simulink subsystem "State_Machine_S1"  (R2023b)
settings: Solver=VariableStepAuto  StartTime=0.0  StopTime=10.0  RelTol=1e-3
undefined symbols (not defined in the file): lb, nF, ub
libraries: dspstat3 x1
settings Model: Creator=Inver  LastModifiedBy=Inver

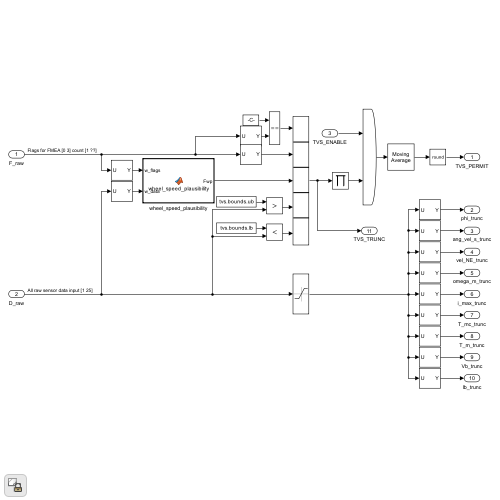
[thumbnail: Simulink's stored preview of the top-level diagram]
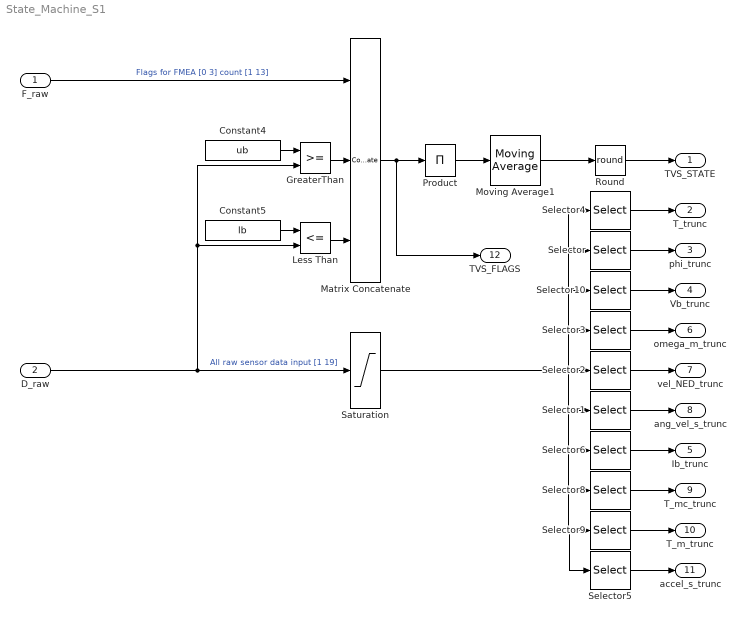
== system State_Machine_S1 ==
  F_raw : Inport
  D_raw : Inport  Port=2
  Constant4 : Constant  Value=ub
  Constant5 : Constant  Value=lb
  GreaterThan : RelationalOperator  OutDataTypeStr=boolean  RndMeth=Simplest  InputSameDT=off
  Less Than : RelationalOperator  Operator=<=  OutDataTypeStr=boolean  RndMeth=Simplest  InputSameDT=off
  Matrix Concatenate : Concatenate  NumInputs=3  ConcatenateDimension=2
  Moving Average1 : dspstat3/Moving Average  Method=Sliding window  ForgettingFactorPort=off  SpecifyWindowLength=on  WindowLength=nF  OverlapLength=nF-1  AllowArbitraryInputLength=off  ForgettingFactor=0.9  SimulateUsing=Code generation
  Product : Product  Inputs=1  OutDataTypeStr=double  SaturateOnIntegerOverflow=on
  Round : Rounding  Operator=round
  Saturation : Saturate  UpperLimit=ub  LowerLimit=lb
  Selector : Selector  IndexMode=Zero-based  InputPortWidth=19  IndexOptions=Index vector (dialog)  Indices=1  OutputSizes=1
  Selector1 : Selector  IndexMode=Zero-based  InputPortWidth=19  IndexOptions=Index vector (dialog)  Indices=[8 9 10]  OutputSizes=1
  Selector10 : Selector  IndexMode=Zero-based  InputPortWidth=19  IndexOptions=Index vector (dialog)  Indices=2  OutputSizes=1
  Selector2 : Selector  IndexMode=Zero-based  InputPortWidth=19  IndexOptions=Index vector (dialog)  Indices=[5 6 7]  OutputSizes=1
  Selector3 : Selector  IndexMode=Zero-based  InputPortWidth=19  IndexOptions=Index vector (dialog)  Indices=[3 4]  OutputSizes=1
  Selector4 : Selector  IndexMode=Zero-based  InputPortWidth=19  IndexOptions=Index vector (dialog)  Indices=0  OutputSizes=1
  Selector5 : Selector  IndexMode=Zero-based  InputPortWidth=19  IndexOptions=Index vector (dialog)  Indices=[16 17 18]  OutputSizes=1
  Selector6 : Selector  IndexMode=Zero-based  InputPortWidth=19  IndexOptions=Index vector (dialog)  Indices=11  OutputSizes=1
  Selector8 : Selector  IndexMode=Zero-based  InputPortWidth=19  IndexOptions=Index vector (dialog)  Indices=[12 13]  OutputSizes=1
  Selector9 : Selector  IndexMode=Zero-based  InputPortWidth=19  IndexOptions=Index vector (dialog)  Indices=[14 15]  OutputSizes=1
  TVS_STATE : Outport
  T_trunc : Outport  Port=2
  phi_trunc : Outport  Port=3
  Vb_trunc : Outport  Port=4
  Ib_trunc : Outport  Port=5
  omega_m_trunc : Outport  Port=6
  vel_NED_trunc : Outport  Port=7
  ang_vel_s_trunc : Outport  Port=8
  T_mc_trunc : Outport  Port=9
  T_m_trunc : Outport  Port=10
  accel_s_trunc : Outport  Port=11
  TVS_FLAGS : Outport  Port=12
  wires:
  Matrix Concatenate/1 -> TVS_FLAGS/1, Product/1
  Round/1 -> TVS_STATE/1
  Selector8/1 -> T_mc_trunc/1
  Selector9/1 -> T_m_trunc/1
  Selector10/1 -> Vb_trunc/1
  Selector6/1 -> Ib_trunc/1
  Selector3/1 -> omega_m_trunc/1
  Selector2/1 -> vel_NED_trunc/1
  Selector1/1 -> ang_vel_s_trunc/1
  Selector/1 -> phi_trunc/1
  Saturation/1 -> Selector3/1, Selector/1, Selector4/1, Selector10/1, Selector2/1, Selector1/1, Selector6/1, Selector8/1, Selector9/1, Selector5/1
  Moving Average1/1 -> Round/1
  Product/1 -> Moving Average1/1
  D_raw/1 -> Less Than/2, GreaterThan/2, Saturation/1  "All raw sensor data input [1 19]"
  Constant5/1 -> Less Than/1
  Constant4/1 -> GreaterThan/1
  GreaterThan/1 -> Matrix Concatenate/2
  Less Than/1 -> Matrix Concatenate/3
  F_raw/1 -> Matrix Concatenate/1  "Flags for FMEA [0 3] count [1 13]"
  Selector4/1 -> T_trunc/1
  Selector5/1 -> accel_s_trunc/1
